simulink model "CHANGE_TL"  (Simulink 6.0)
settings: Solver=ode45  StartTime=0.0  StopTime=10  RelTol=1e-3
settings Model: LastModifiedBy=John

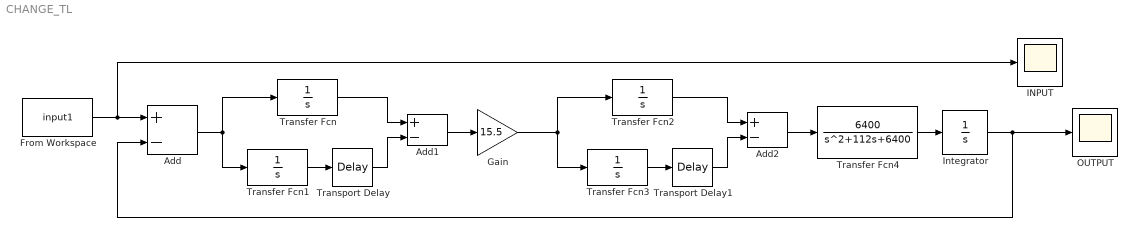
== system CHANGE_TL ==
  Add : Sum  Inputs=+-  OutScaling=2^-10
  Add1 : Sum  Inputs=+-  OutScaling=2^-10
  Add2 : Sum  Inputs=+-  OutScaling=2^-10
  From Workspace : FromWorkspace  VariableName=input1  SampleTime=0
  Gain : Gain  Gain=15.5
  INPUT : Scope
      settings: SaveName=INPUT  DataFormat=Array
  Integrator : Integrator
  OUTPUT : Scope
      settings: SaveName=OUTPUT  DataFormat=Array
  Transfer Fcn{,1..3} (4 alike) : TransferFcn  Denominator=[1 0]
  Transfer Fcn4 : TransferFcn  Numerator=[6400]  Denominator=[1 112 6400]
  Transport Delay : TransportDelay  DelayTime=1.4
  Transport Delay1 : TransportDelay  DelayTime=0.04
  wires:
  Add/1 -> Transfer Fcn/1, Transfer Fcn1/1
  From Workspace/1 -> Add/1, INPUT/1
  Transfer Fcn/1 -> Add1/1
  Transfer Fcn4/1 -> Integrator/1
  Integrator/1 -> Add/2, OUTPUT/1
  Transfer Fcn1/1 -> Transport Delay/1
  Transport Delay/1 -> Add1/2
  Add1/1 -> Gain/1
  Gain/1 -> Transfer Fcn2/1, Transfer Fcn3/1
  Transfer Fcn2/1 -> Add2/1
  Add2/1 -> Transfer Fcn4/1
  Transfer Fcn3/1 -> Transport Delay1/1
  Transport Delay1/1 -> Add2/2
